simulink model "Target"  (R2013a)
settings: Solver=FixedStepDiscrete  StartTime=0.0  StopTime=10.0  RelTol=1e-3
undefined symbols (not defined in the file or in its folder): Link1, Link2, Link3, Link4, Link5, Link6
libraries: vrlib x3, dspnetwork x2, linuxlib x1
settings Model: Creator=rkaria  LastModifiedBy=rkaria
settings OptimizationCC: OptimizeModelRefInitCode=on  LifeSpan=1
settings HardwareCC: ProdIntDivRoundTo=Zero  ProdEndianess=LittleEndian  ProdHWDeviceType=Intel->x86/Pentium
settings RTWCC: SystemTargetFile=ert.tlc  GenCodeOnly=on  TemplateMakefile=ert_default_tmf  Description=Embedded Coder  GenerateReport=on  ProcessScript=ert_make_rtw_hook  IncludeHyperlinkInReport=on  LaunchReport=on
settings CodeAppCC: IgnoreCustomStorageClasses=off
settings ERTTargetCC: InlinedParameterPlacement=Hierarchical  ERTCustomFileTemplate=example_file_process.tlc

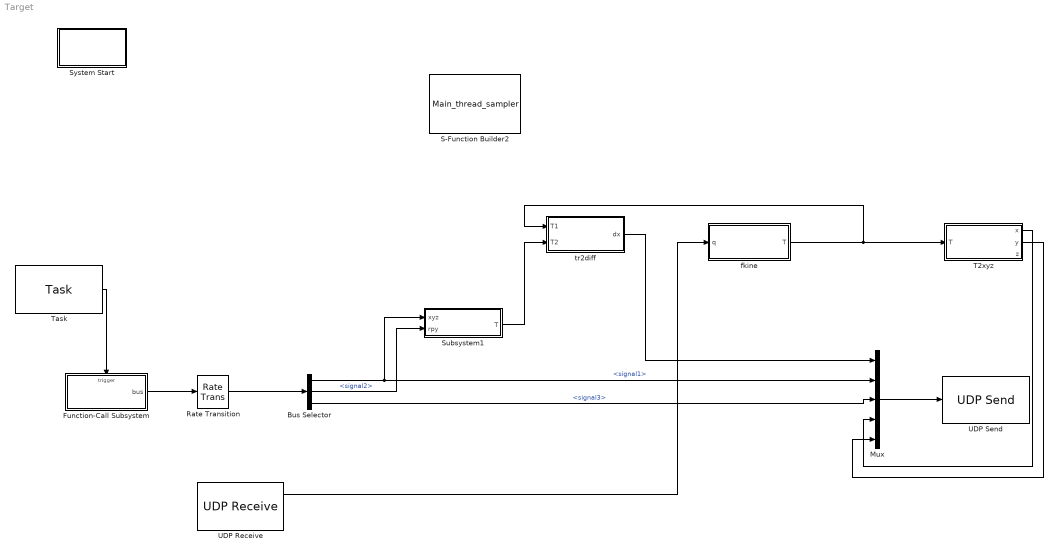
== system Target ==
  Bus Selector : BusSelector
  Function-Call Subsystem : Subsystem  Priority=2  TreatAsAtomicUnit=on
  Mux : Mux  Inputs=5
  Rate Transition : RateTransition  Deterministic=off  OutPortSampleTimeOpt=Inherit
  S-Function Builder2 : S-Function  Priority=1  InitFcn=try, set_param(gcb,'FunctionName','Main_thread_sampler'), end  FunctionName=Main_thread_sampler  SFunctionModules=Main_thread_sampler_wrapper  EnableBusSupport=off  mask(S-Function Builder){}
      mask help: Simulink:masks:SFunctionBuilder_MD
      mask init:
      | val = [[.9  0.75 0.75 1 1 .9 .9 1]',[1 1 0.75 0.75 .9 .9 1 .9]'];try , sys = get_param(gcb,'SfunBuilderFcnName');if isempty(sys), sys = get_param(gcb,'FunctionName'); end,catch, sys = get_param(gcb,'FunctionName'); end
      settings: CopyFcn=set_param(gcbh,'LinkStatus','none')  PreSaveFcn=try, set_param(gcb,'FunctionName','Main_thread_sampler'), end  OpenFcn=sfunctionwizard(gcbh)
      mask Display:
      | plot(val(:,1),val(:,2))
      | disp(sys)
  Subsystem1 : Subsystem
  System Start : Subsystem  mask(System Start){ShowInLibBrowser=0}
      mask prompts: ShowInLibBrowser "Simulink:masks:CustCodeMaskParam1_MP"
      settings: CopyFcn=cccopyfcn(gcb)  OpenFcn=ccopenfcn('System Start Function')
      mask Help: eval('feval(''rtwprivate'',''rtwhelpview'',''rtw_sys_start_block'')');
      mask Display: disp('System\nStart');
  T2xyz : Subsystem
  Task : linuxlib/Task  Priority=2  taskName=Task0  taskPolicy=SCHED_FIFO  taskPriority=1
  UDP Receive : dspnetwork/UDP Receive  localURL='0.0.0.0'  localPort=25001  remoteURL='0.0.0.0'  remotePort=-1  recvBufferSize=8192  dims=6  signalDatatype=double  isVarSize=off  showBlockingTime=on  blockingTime=0.7  sampletime=-1  blockPlatform=LINUX
  UDP Send : dspnetwork/UDP Send  remoteURL='10.218.99.202'  remotePort=25000  localURL='255.255.255.255'  localPortSource=Automatically determine  localPort=-1  sampletime=-1  blockPlatform=LINUX  separateLengthPort=0
  fkine : Subsystem  TreatAsAtomicUnit=on
  tr2diff : Subsystem
  wires:
  Task/1 -> Function-Call Subsystem/Trigger
  Function-Call Subsystem/1(bus) -> Rate Transition/1
  fkine/1(T) -> T2xyz/1(T), tr2diff/1(T1)
  Subsystem1/1(T) -> tr2diff/2(T2)
  Rate Transition/1 -> Bus Selector/1
  Bus Selector/1 -> Subsystem1/1(xyz), Mux/2  "<signal1>"
  Bus Selector/2 -> Subsystem1/2(rpy)  "<signal2>"
  Bus Selector/3 -> Mux/3  "<signal3>"
  tr2diff/1(dx) -> Mux/1
  T2xyz/1(x) -> Mux/4
  T2xyz/2(y) -> Mux/5
  Mux/1 -> UDP Send/1
  UDP Receive/1 -> fkine/1(q)

== system Target/Function-Call Subsystem ==
  function : TriggerPort  TriggerType=function-call
  Bus Creator : BusCreator  Inputs=3
  Trajectory generation1 : Subsystem
  bus : Outport
  wires:
  Trajectory generation1/1(xyz) -> Bus Creator/1
  Trajectory generation1/2(rpy) -> Bus Creator/2
  Trajectory generation1/3(clear) -> Bus Creator/3
  Bus Creator/1 -> bus/1

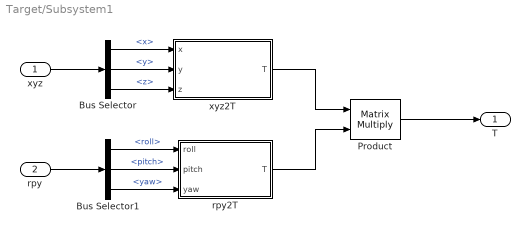
== system Target/Subsystem1 ==
  xyz : Inport
  rpy : Inport  Port=2
  Bus Selector : BusSelector  OutputSignals=x,y,z
  Bus Selector1 : BusSelector  OutputSignals=roll,pitch,yaw
  Product : Product  Multiplication=Matrix(*)  RndMeth=Zero
  rpy2T : Subsystem
  xyz2T : Subsystem
  T : Outport
  wires:
  xyz/1 -> Bus Selector/1
  Bus Selector/1 -> xyz2T/1(x)  "<x>"
  Bus Selector/2 -> xyz2T/2(y)  "<y>"
  Bus Selector/3 -> xyz2T/3(z)  "<z>"
  xyz2T/1(T) -> Product/1
  Product/1 -> T/1
  rpy2T/1(T) -> Product/2
  rpy/1 -> Bus Selector1/1
  Bus Selector1/1 -> rpy2T/1(roll)  "<roll>"
  Bus Selector1/2 -> rpy2T/2(pitch)  "<pitch>"
  Bus Selector1/3 -> rpy2T/3(yaw)  "<yaw>"

== system Target/System Start ==

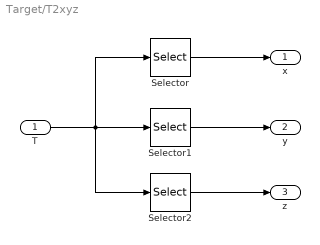
== system Target/T2xyz ==
  T : Inport
  Selector : Selector  NumberOfDimensions=2  InputPortWidth=3  IndexOptions=Index vector (dialog),Index vector (dialog)  Indices=1,4  OutputSizes=1,1
  Selector1 : Selector  NumberOfDimensions=2  InputPortWidth=3  IndexOptions=Index vector (dialog),Index vector (dialog)  Indices=2,4  OutputSizes=1,1
  Selector2 : Selector  NumberOfDimensions=2  InputPortWidth=3  IndexOptions=Index vector (dialog),Index vector (dialog)  Indices=3,4  OutputSizes=1,1
  x : Outport
  y : Outport  Port=2
  z : Outport  Port=3
  wires:
  Selector/1 -> x/1
  Selector1/1 -> y/1
  Selector2/1 -> z/1
  T/1 -> Selector/1, Selector2/1, Selector1/1

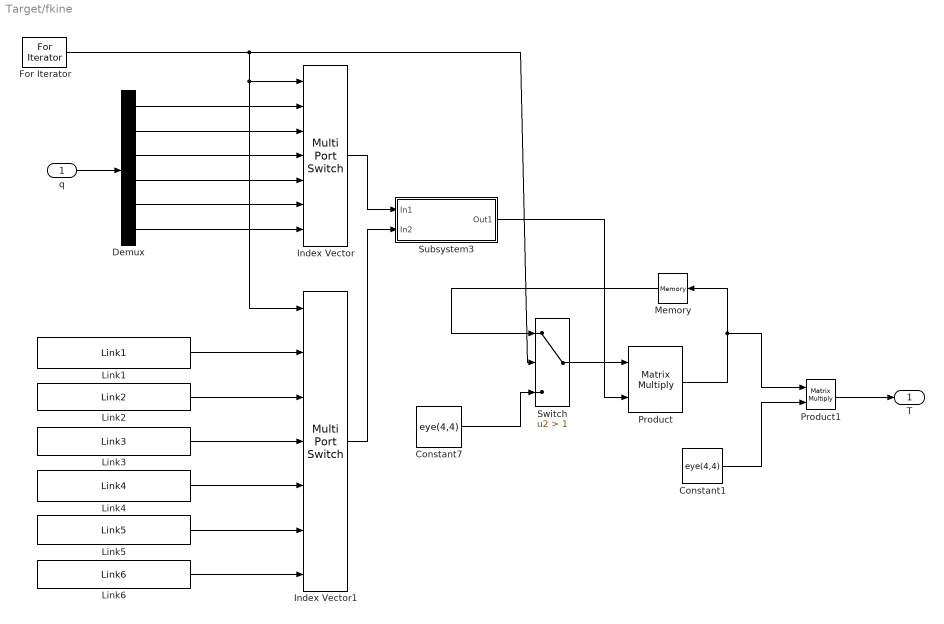
== system Target/fkine ==
  q : Inport
  Constant1 : Constant  Value=eye(4,4)
  Constant7 : Constant  Value=eye(4,4)
  Demux : Demux  Outputs=6
  For Iterator : ForIterator  IterationLimit=NoOfLinks
  Index Vector : MultiPortSwitch  Inputs=6
  Index Vector1 : MultiPortSwitch  Inputs=6
  Link1 : Constant  Value=Link1
  Link2 : Constant  Value=Link2
  Link3 : Constant  Value=Link3
  Link4 : Constant  Value=Link4
  Link5 : Constant  Value=Link5
  Link6 : Constant  Value=Link6
  Memory : Memory  X0=eye(4,4)  InheritSampleTime=on
  Product : Product  Multiplication=Matrix(*)  RndMeth=Zero
  Product1 : Product  Multiplication=Matrix(*)  RndMeth=Zero
  Subsystem3 : Subsystem
  Switch : Switch  Criteria=u2 > Threshold  Threshold=1
  T : Outport
  wires:
  Memory/1 -> Switch/1
  Switch/1 -> Product/1
  Subsystem3/1(Out1) -> Product/2
  Constant7/1 -> Switch/3
  Product/1 -> Product1/1, Memory/1
  Index Vector1/1 -> Subsystem3/2(In2)
  Index Vector/1 -> Subsystem3/1(In1)
  Demux/6 -> Index Vector/7
  Demux/5 -> Index Vector/6
  Demux/4 -> Index Vector/5
  Demux/3 -> Index Vector/4
  Demux/2 -> Index Vector/3
  Demux/1 -> Index Vector/2
  q/1 -> Demux/1
  Link6/1 -> Index Vector1/7
  Link5/1 -> Index Vector1/6
  Link4/1 -> Index Vector1/5
  Link3/1 -> Index Vector1/4
  Link2/1 -> Index Vector1/3
  Link1/1 -> Index Vector1/2
  For Iterator/1 -> Switch/2, Index Vector1/1, Index Vector/1
  Product1/1 -> T/1
  Constant1/1 -> Product1/2

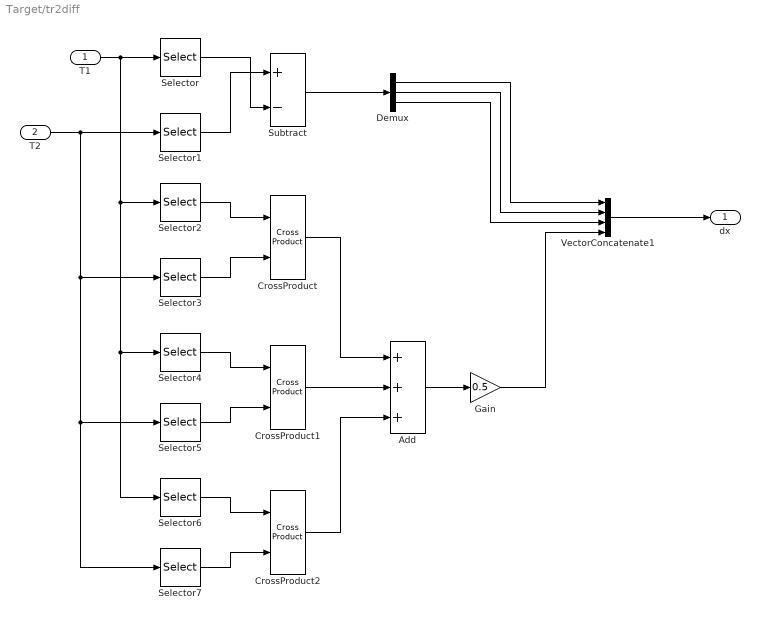
== system Target/tr2diff ==
  T1 : Inport
  T2 : Inport  Port=2
  Add : Sum  Inputs=+++
  CrossProduct : vrlib/Utilities/Cross Product
  CrossProduct1 : vrlib/Utilities/Cross Product
  CrossProduct2 : vrlib/Utilities/Cross Product
  Demux : Demux  Outputs=3
  Gain : Gain  Gain=0.5
  Selector : Selector  NumberOfDimensions=2  InputPortWidth=3  IndexOptions=Index vector (dialog),Index vector (dialog)  Indices=[1:3],4  OutputSizes=1,1
  Selector1 : Selector  NumberOfDimensions=2  InputPortWidth=3  IndexOptions=Index vector (dialog),Index vector (dialog)  Indices=[1:3],4  OutputSizes=1,1
  Selector2 : Selector  NumberOfDimensions=2  InputPortWidth=3  IndexOptions=Index vector (dialog),Index vector (dialog)  Indices=[1:3],1  OutputSizes=1,1
  Selector3 : Selector  NumberOfDimensions=2  InputPortWidth=3  IndexOptions=Index vector (dialog),Index vector (dialog)  Indices=[1:3],1  OutputSizes=1,1
  Selector4 : Selector  NumberOfDimensions=2  InputPortWidth=3  IndexOptions=Index vector (dialog),Index vector (dialog)  Indices=[1:3],2  OutputSizes=1,1
  Selector5 : Selector  NumberOfDimensions=2  InputPortWidth=3  IndexOptions=Index vector (dialog),Index vector (dialog)  Indices=[1:3],2  OutputSizes=1,1
  Selector6 : Selector  NumberOfDimensions=2  InputPortWidth=3  IndexOptions=Index vector (dialog),Index vector (dialog)  Indices=[1:3],3  OutputSizes=1,1
  Selector7 : Selector  NumberOfDimensions=2  InputPortWidth=3  IndexOptions=Index vector (dialog),Index vector (dialog)  Indices=[1:3],3  OutputSizes=1,1
  Subtract : Sum  Inputs=+-
  VectorConcatenate1 : Concatenate  NumInputs=4
  dx : Outport
  wires:
  T1/1 -> Selector/1, Selector2/1, Selector6/1, Selector4/1
  T2/1 -> Selector1/1, Selector7/1, Selector5/1, Selector3/1
  Selector1/1 -> Subtract/1
  Selector/1 -> Subtract/2
  Selector2/1 -> CrossProduct/1
  Selector3/1 -> CrossProduct/2
  Selector4/1 -> CrossProduct1/1
  Selector5/1 -> CrossProduct1/2
  Selector6/1 -> CrossProduct2/1
  Selector7/1 -> CrossProduct2/2
  CrossProduct/1 -> Add/1
  CrossProduct1/1 -> Add/2
  CrossProduct2/1 -> Add/3
  Add/1 -> Gain/1
  VectorConcatenate1/1 -> dx/1
  Subtract/1 -> Demux/1
  Demux/1 -> VectorConcatenate1/1
  Demux/2 -> VectorConcatenate1/2
  Demux/3 -> VectorConcatenate1/3
  Gain/1 -> VectorConcatenate1/4

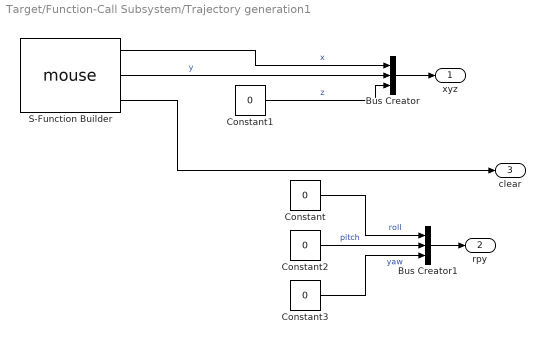
== system Target/Function-Call Subsystem/Trajectory generation1 ==
  Bus Creator : BusCreator  Inputs='x','y','z'
  Bus Creator1 : BusCreator  Inputs=3
  Constant : Constant  Value=0  VectorParams1D=off
  Constant1 : Constant  Value=0
  Constant2 : Constant  Value=0
  Constant3 : Constant  Value=0
  S-Function Builder : S-Function  InitFcn=try, set_param(gcb,'FunctionName','mouse'), end  FunctionName=mouse  SFunctionModules=mouse_wrapper  EnableBusSupport=off  mask(S-Function Builder){}
      mask help: Simulink:masks:SFunctionBuilder_MD
      mask init: same as Target/S-Function Builder2
      settings: CopyFcn=set_param(gcbh,'LinkStatus','none')  PreSaveFcn=try, set_param(gcb,'FunctionName','mouse'), end  OpenFcn=sfunctionwizard(gcbh)
      mask Display: plot(val(:,1),val(:,2)),disp(sys), port_label('output',1,'SCALED_X'), port_label('output',2,'SCALED_Y'), port_label('output',3,'CLEAR')
  xyz : Outport
  rpy : Outport  Port=2
  clear : Outport  Port=3
  wires:
  Constant1/1 -> Bus Creator/3  "z"
  Bus Creator/1 -> xyz/1
  Constant2/1 -> Bus Creator1/2  "pitch"
  Constant/1 -> Bus Creator1/1  "roll"
  Constant3/1 -> Bus Creator1/3  "yaw"
  Bus Creator1/1 -> rpy/1
  S-Function Builder/1 -> Bus Creator/1  "x"
  S-Function Builder/2 -> Bus Creator/2  "y"
  S-Function Builder/3 -> clear/1

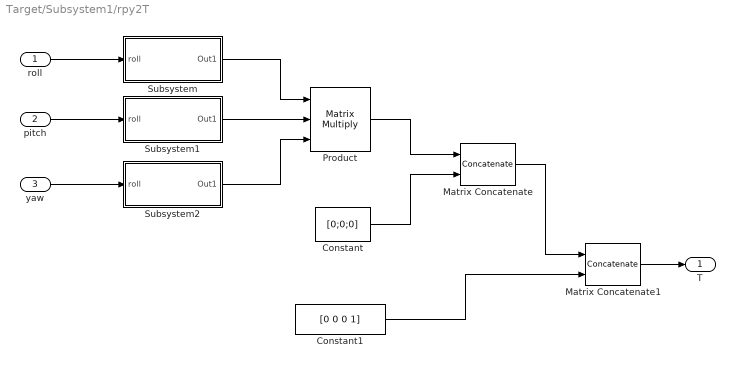
== system Target/Subsystem1/rpy2T ==
  roll : Inport
  pitch : Inport  Port=2
  yaw : Inport  Port=3
  Constant : Constant  Value=[0;0;0]
  Constant1 : Constant  Value=[0 0 0 1]  VectorParams1D=off
  Matrix Concatenate : Concatenate  Mode=Multidimensional array  ConcatenateDimension=2
  Matrix Concatenate1 : Concatenate  Mode=Multidimensional array
  Product : Product  Inputs=3  Multiplication=Matrix(*)  RndMeth=Zero
  Subsystem : Subsystem
  Subsystem1 : Subsystem
  Subsystem2 : Subsystem
  T : Outport
  wires:
  roll/1 -> Subsystem/1(roll)
  pitch/1 -> Subsystem1/1(roll)
  yaw/1 -> Subsystem2/1(roll)
  Subsystem/1(Out1) -> Product/1
  Subsystem1/1(Out1) -> Product/2
  Subsystem2/1(Out1) -> Product/3
  Product/1 -> Matrix Concatenate/1
  Constant/1 -> Matrix Concatenate/2
  Matrix Concatenate/1 -> Matrix Concatenate1/1
  Constant1/1 -> Matrix Concatenate1/2
  Matrix Concatenate1/1 -> T/1

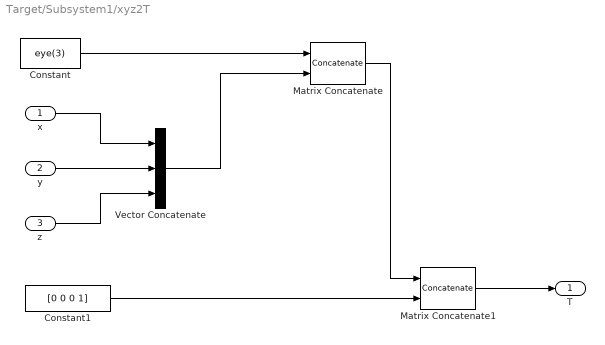
== system Target/Subsystem1/xyz2T ==
  x : Inport
  y : Inport  Port=2
  z : Inport  Port=3
  Constant : Constant  Value=eye(3)
  Constant1 : Constant  Value=[0 0 0 1]  VectorParams1D=off
  Matrix Concatenate : Concatenate  Mode=Multidimensional array  ConcatenateDimension=2
  Matrix Concatenate1 : Concatenate  Mode=Multidimensional array
  Vector Concatenate : Concatenate  NumInputs=3
  T : Outport
  wires:
  x/1 -> Vector Concatenate/1
  y/1 -> Vector Concatenate/2
  z/1 -> Vector Concatenate/3
  Constant/1 -> Matrix Concatenate/1
  Vector Concatenate/1 -> Matrix Concatenate/2
  Matrix Concatenate/1 -> Matrix Concatenate1/1
  Constant1/1 -> Matrix Concatenate1/2
  Matrix Concatenate1/1 -> T/1

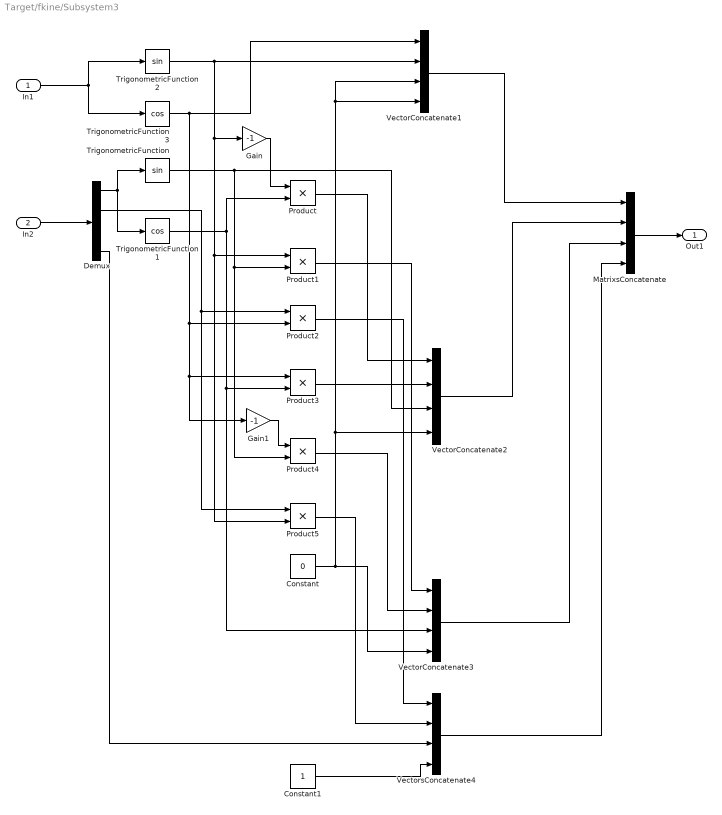
== system Target/fkine/Subsystem3 ==
  In1 : Inport
  In2 : Inport  Port=2
  Constant : Constant  Value=0
  Constant1 : Constant
  Demux : Demux
  Gain : Gain  Gain=-1
  Gain1 : Gain  Gain=-1
  MatrixsConcatenate : Concatenate  NumInputs=4  Mode=Multidimensional array  ConcatenateDimension=2
  Product{,1..5} (6 alike) : Product  RndMeth=Zero
  TrigonometricFunction : Trigonometry
  TrigonometricFunction1 : Trigonometry  Operator=cos
  TrigonometricFunction2 : Trigonometry
  TrigonometricFunction3 : Trigonometry  Operator=cos
  VectorConcatenate1 : Concatenate  NumInputs=4  ConcatenateDimension=2
  VectorConcatenate2 : Concatenate  NumInputs=4  ConcatenateDimension=2
  VectorConcatenate3 : Concatenate  NumInputs=4  ConcatenateDimension=2
  VectorsConcatenate4 : Concatenate  NumInputs=4  ConcatenateDimension=2
  Out1 : Outport
  wires:
  VectorsConcatenate4/1 -> MatrixsConcatenate/4
  VectorConcatenate3/1 -> MatrixsConcatenate/3
  VectorConcatenate2/1 -> MatrixsConcatenate/2
  VectorConcatenate1/1 -> MatrixsConcatenate/1
  MatrixsConcatenate/1 -> Out1/1
  Constant1/1 -> VectorsConcatenate4/4
  Constant/1 -> VectorConcatenate1/3, VectorConcatenate1/4, VectorConcatenate2/4, VectorConcatenate3/4
  Gain1/1 -> Product4/1
  Product3/1 -> VectorConcatenate2/2
  Demux/2 -> Product5/1, Product2/1
  TrigonometricFunction/1 -> Product1/2, Product4/2, VectorConcatenate2/3
  TrigonometricFunction3/1 -> VectorConcatenate1/1, Gain1/1, Product3/1, Product2/2
  TrigonometricFunction1/1 -> VectorConcatenate3/3, Product3/2, Product/2
  Gain/1 -> Product/1
  TrigonometricFunction2/1 -> Product5/2, Product1/1, Gain/1, VectorConcatenate1/2
  Demux/1 -> TrigonometricFunction1/1, TrigonometricFunction/1
  In1/1 -> TrigonometricFunction3/1, TrigonometricFunction2/1
  In2/1 -> Demux/1
  Product/1 -> VectorConcatenate2/1
  Product4/1 -> VectorConcatenate3/2
  Product1/1 -> VectorConcatenate3/1
  Product2/1 -> VectorsConcatenate4/1
  Product5/1 -> VectorsConcatenate4/2
  Demux/4 -> VectorsConcatenate4/3

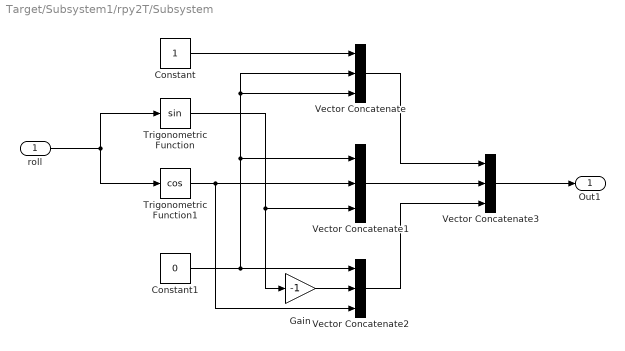
== system Target/Subsystem1/rpy2T/Subsystem ==
  roll : Inport
  Constant : Constant
  Constant1 : Constant  Value=0
  Gain : Gain  Gain=-1
  Trigonometric Function : Trigonometry
  Trigonometric Function1 : Trigonometry  Operator=cos
  Vector Concatenate : Concatenate  NumInputs=3
  Vector Concatenate1 : Concatenate  NumInputs=3
  Vector Concatenate2 : Concatenate  NumInputs=3
  Vector Concatenate3 : Concatenate  NumInputs=3  Mode=Multidimensional array  ConcatenateDimension=2
  Out1 : Outport
  wires:
  roll/1 -> Trigonometric Function/1, Trigonometric Function1/1
  Constant/1 -> Vector Concatenate/1
  Trigonometric Function1/1 -> Vector Concatenate1/2, Vector Concatenate2/3
  Trigonometric Function/1 -> Gain/1, Vector Concatenate1/3
  Vector Concatenate/1 -> Vector Concatenate3/1
  Vector Concatenate1/1 -> Vector Concatenate3/2
  Vector Concatenate2/1 -> Vector Concatenate3/3
  Constant1/1 -> Vector Concatenate/2, Vector Concatenate/3, Vector Concatenate1/1, Vector Concatenate2/1
  Gain/1 -> Vector Concatenate2/2
  Vector Concatenate3/1 -> Out1/1

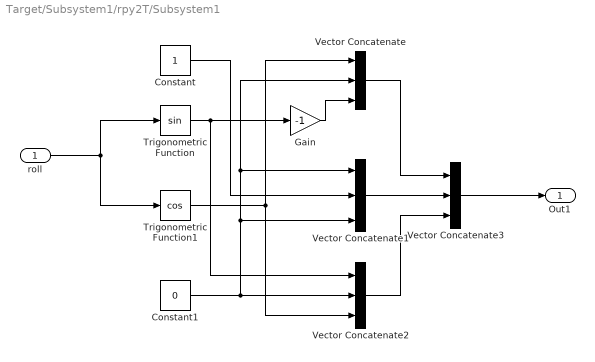
== system Target/Subsystem1/rpy2T/Subsystem1 ==
  roll : Inport
  Constant : Constant
  Constant1 : Constant  Value=0
  Gain : Gain  Gain=-1
  Trigonometric Function : Trigonometry
  Trigonometric Function1 : Trigonometry  Operator=cos
  Vector Concatenate : Concatenate  NumInputs=3
  Vector Concatenate1 : Concatenate  NumInputs=3
  Vector Concatenate2 : Concatenate  NumInputs=3
  Vector Concatenate3 : Concatenate  NumInputs=3  Mode=Multidimensional array  ConcatenateDimension=2
  Out1 : Outport
  wires:
  roll/1 -> Trigonometric Function/1, Trigonometric Function1/1
  Vector Concatenate/1 -> Vector Concatenate3/1
  Vector Concatenate1/1 -> Vector Concatenate3/2
  Vector Concatenate2/1 -> Vector Concatenate3/3
  Trigonometric Function1/1 -> Vector Concatenate/1, Vector Concatenate2/3
  Constant1/1 -> Vector Concatenate2/2, Vector Concatenate/2, Vector Concatenate1/1, Vector Concatenate1/3
  Trigonometric Function/1 -> Gain/1, Vector Concatenate2/1
  Constant/1 -> Vector Concatenate1/2
  Gain/1 -> Vector Concatenate/3
  Vector Concatenate3/1 -> Out1/1

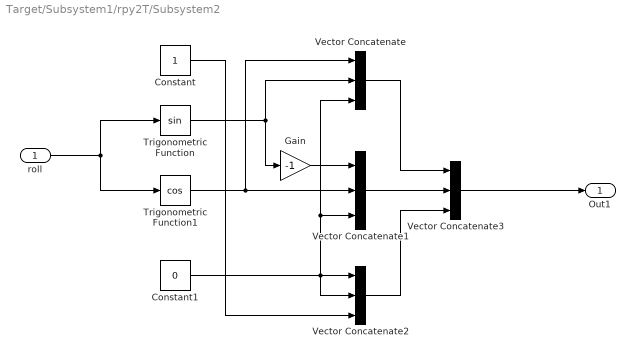
== system Target/Subsystem1/rpy2T/Subsystem2 ==
  roll : Inport
  Constant : Constant
  Constant1 : Constant  Value=0
  Gain : Gain  Gain=-1
  Trigonometric Function : Trigonometry
  Trigonometric Function1 : Trigonometry  Operator=cos
  Vector Concatenate : Concatenate  NumInputs=3
  Vector Concatenate1 : Concatenate  NumInputs=3
  Vector Concatenate2 : Concatenate  NumInputs=3
  Vector Concatenate3 : Concatenate  NumInputs=3  Mode=Multidimensional array  ConcatenateDimension=2
  Out1 : Outport
  wires:
  roll/1 -> Trigonometric Function/1, Trigonometric Function1/1
  Vector Concatenate/1 -> Vector Concatenate3/1
  Vector Concatenate1/1 -> Vector Concatenate3/2
  Vector Concatenate2/1 -> Vector Concatenate3/3
  Trigonometric Function1/1 -> Vector Concatenate/1, Vector Concatenate1/2
  Trigonometric Function/1 -> Vector Concatenate/2, Gain/1
  Constant1/1 -> Vector Concatenate/3, Vector Concatenate1/3, Vector Concatenate2/1, Vector Concatenate2/2
  Constant/1 -> Vector Concatenate2/3
  Gain/1 -> Vector Concatenate1/1
  Vector Concatenate3/1 -> Out1/1
